simulink model "ModularDBIPSimulation"  (R2025a)
settings: Solver=FixedStepAuto  StartTime=0.0  StopTime=60  FixedStep=0.001  RelTol=1e-3
values from neighbouring files (symbols this model uses):
  A_linearized_numeric = double(subs(A_linearized,model_params,param_values))    [DBIP_CtrlStrategies.m]
  Ac = [Ac1 zeros(1,6);Ac3 Ac2]    [DBIP_CtrlStrategies.m]
  Ao = M    [DBIP_CtrlStrategies.m]
  B_linearized_numeric = double(subs(B_linearized,model_params,param_values))    [DBIP_CtrlStrategies.m]
  Bc = [Bc1;Bc2]    [DBIP_CtrlStrategies.m]
  Bo = [N P]    [DBIP_CtrlStrategies.m]
  C = eye(6)    [DBIP_SymbolicDerivation.m]
  Cc = [Cc1 Cc2]    [DBIP_CtrlStrategies.m]
  Co = Q    [DBIP_CtrlStrategies.m]
  D = [0, 0, 0, 0, 0, 0].'    [DBIP_SymbolicDerivation.m]
  Dc = zeros(1,4)    [DBIP_CtrlStrategies.m]
  Do = [R S]    [DBIP_CtrlStrategies.m]
  F = [F1 F2]    [DBIP_CtrlStrategies.m]
  theta_ref = input('Enter the desired reference theta (deg):')    [DBIP_CtrlStrategies.m]
  x0 = [deg2rad(theta_i); deg2rad(alpha_i); deg2rad(phi_i); 0; 0; 0]    [DBIP_CtrlStrategies.m]
  x2_ref = deg2rad(theta_desired)    [DBIP_CtrlStrategies.m]
  xc_o = [deg2rad(theta_i); deg2rad(alpha_i); deg2rad(phi_i); 0; 0;0;deg2rad(theta_ref)]    [DBIP_CtrlStrategies.m]
  z_o = L*(C1^-1)*y_o    [DBIP_CtrlStrategies.m]
libraries: simulink_extras x2
settings Model: Creator=young  LastModifiedBy=young
settings DataIOCC: ReturnWorkspaceOutputs=off
settings DebuggingCC: AlgebraicLoopMsg=none

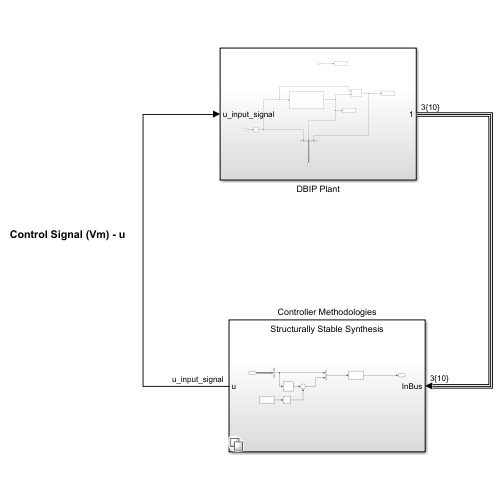
[thumbnail: Simulink's stored preview of the top-level diagram]
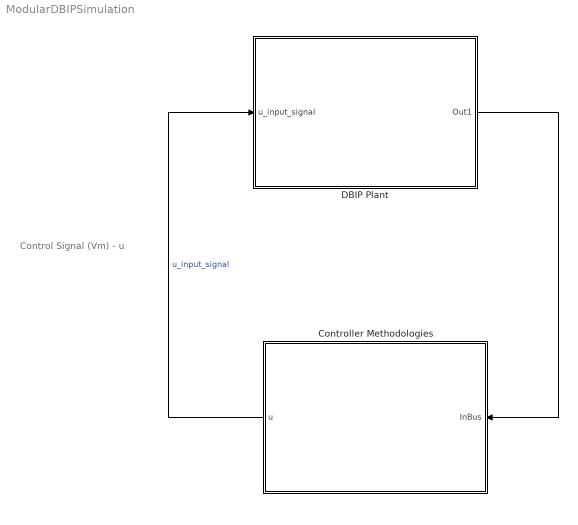
== system ModularDBIPSimulation ==
  note: Control Signal (Vm) - u
  Controller Methodologies : Subsystem  Variant=on
  DBIP Plant : Subsystem
  wires:
  Controller Methodologies/1(u) -> DBIP Plant/1(u_input_signal)  "u_input_signal"
  DBIP Plant/1(Out1) -> Controller Methodologies/1(InBus)

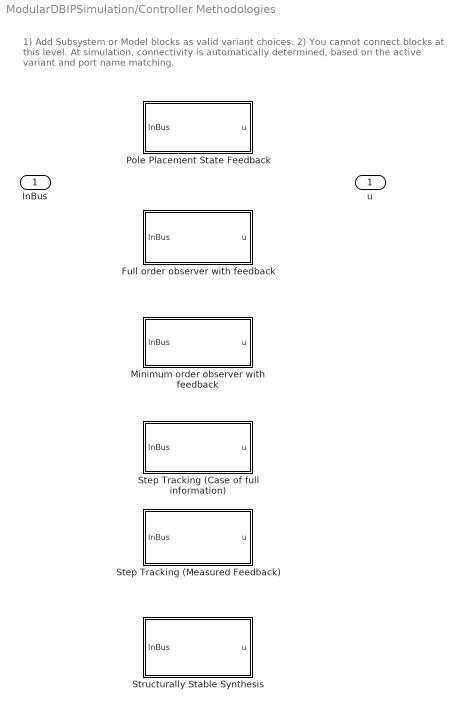
== system ModularDBIPSimulation/Controller Methodologies ==
  note: 1) Add Subsystem or Model blocks as valid variant choices.
      | 2) You cannot connect blocks at this level. At simulation, connectivity is automatically
      | determined, based on the active variant and port name matching.
  InBus : Inport
  Full order observer with feedback : Subsystem  VariantControl=control_strategy == 2
  Minimum order observer with feedback : Subsystem  VariantControl=control_strategy == 3
  Pole Placement State Feedback : Subsystem  VariantControl=control_strategy == 1
  Step Tracking (Case of full information) : Subsystem  VariantControl=control_strategy == 4
  Step Tracking (Measured Feedback) : Subsystem  VariantControl=control_strategy == 5
  Structurally Stable Synthesis : Subsystem  VariantControl=control_strategy==6
  u : Outport

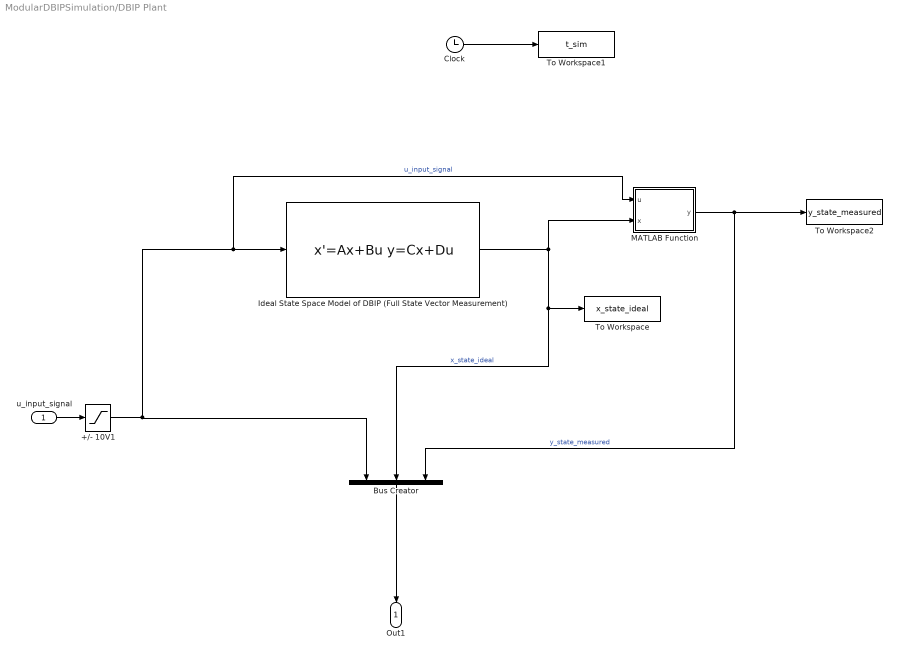
== system ModularDBIPSimulation/DBIP Plant ==
  u_input_signal : Inport
  +/- 10V1 : Saturate  UpperLimit=10  LowerLimit=-10
  Bus Creator : BusCreator  Inputs=3
  Clock : Clock
  Ideal State Space Model of DBIP (Full State Vector Measurement) : StateSpace  A=A_linearized_numeric  B=B_linearized_numeric  C=C  D=D  InitialCondition=x0
  MATLAB Function : MATLAB Function  TreatAsAtomicUnit=on
  To Workspace : ToWorkspace  VariableName=x_state_ideal  SampleTime=-1
  To Workspace1 : ToWorkspace  VariableName=t_sim  SampleTime=-1
  To Workspace2 : ToWorkspace  VariableName=y_state_measured  SampleTime=-1
  Out1 : Outport
  wires:
  MATLAB Function/1(y) -> Bus Creator/3, To Workspace2/1  "y_state_measured"
  u_input_signal/1 -> +/- 10V1/1
  Ideal State Space Model of DBIP (Full State Vector Measurement)/1 -> MATLAB Function/2(x), Bus Creator/2, To Workspace/1  "x_state_ideal"
  Bus Creator/1 -> Out1/1
  Clock/1 -> To Workspace1/1
  +/- 10V1/1 -> Ideal State Space Model of DBIP (Full State Vector Measurement)/1, MATLAB Function/1(u), Bus Creator/1  "u_input_signal"

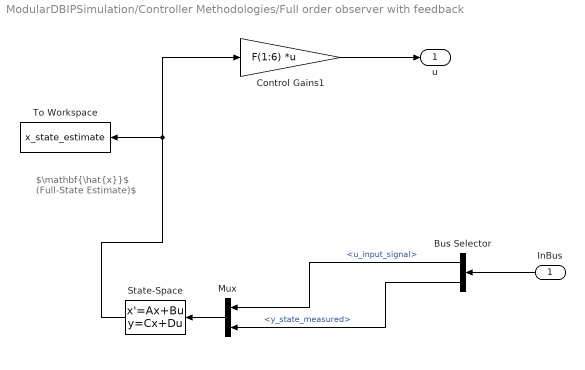
== system ModularDBIPSimulation/Controller Methodologies/Full order observer with feedback ==
  note: $\mathbf{\hat{x}}$ (Full-State Estimate)$
  InBus : Inport
  Bus Selector : BusSelector  OutputSignals=u_input_signal,y_state_measured
  Control Gains1 : Gain  Gain=F(1:6)  Multiplication=Matrix(K*u)
  Mux : Mux  Inputs=2
  State-Space : StateSpace  A=Ao  B=Bo  C=Co  D=Do  InitialCondition=z_o
  To Workspace : ToWorkspace  VariableName=x_state_estimate  SampleTime=-1
  u : Outport
  wires:
  State-Space/1 -> Control Gains1/1, To Workspace/1
  Control Gains1/1 -> u/1
  InBus/1 -> Bus Selector/1
  Bus Selector/1 -> Mux/1  "<u_input_signal>"
  Bus Selector/2 -> Mux/2  "<y_state_measured>"
  Mux/1 -> State-Space/1

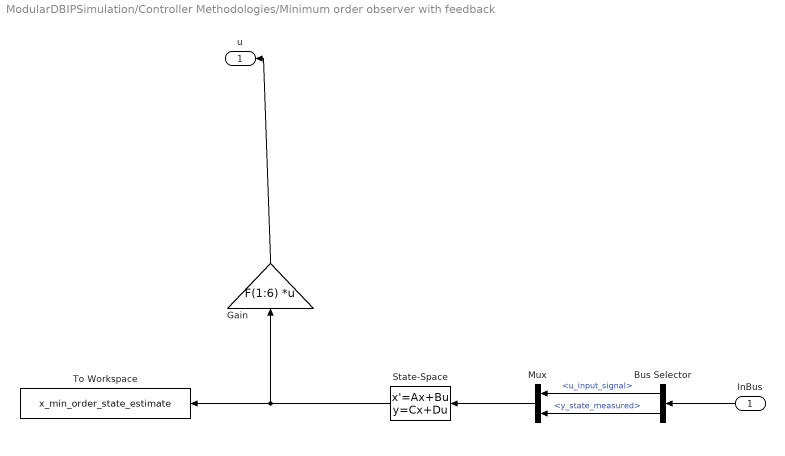
== system ModularDBIPSimulation/Controller Methodologies/Minimum order observer with feedback ==
  InBus : Inport
  Bus Selector : BusSelector  OutputSignals=u_input_signal,y_state_measured
  Gain : Gain  Gain=F(1:6)  Multiplication=Matrix(K*u)
  Mux : Mux  Inputs=2
  State-Space : StateSpace  A=Ao  B=Bo  C=Co  D=Do  InitialCondition=z_o
  To Workspace : ToWorkspace  VariableName=x_min_order_state_estimate  SampleTime=-1
  u : Outport
  wires:
  InBus/1 -> Bus Selector/1
  Gain/1 -> u/1
  State-Space/1 -> To Workspace/1, Gain/1
  Bus Selector/2 -> Mux/2  "<y_state_measured>"
  Bus Selector/1 -> Mux/1  "<u_input_signal>"
  Mux/1 -> State-Space/1

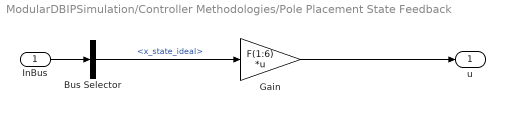
== system ModularDBIPSimulation/Controller Methodologies/Pole Placement State Feedback ==
  InBus : Inport
  Bus Selector : BusSelector  OutputSignals=x_state_ideal
  Gain : Gain  Gain=F(1:6)  Multiplication=Matrix(K*u)
  u : Outport
  wires:
  Gain/1 -> u/1
  InBus/1 -> Bus Selector/1
  Bus Selector/1 -> Gain/1  "<x_state_ideal>"

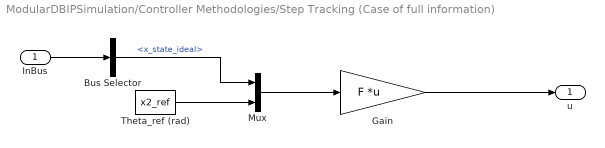
== system ModularDBIPSimulation/Controller Methodologies/Step Tracking (Case of full information) ==
  InBus : Inport
  Bus Selector : BusSelector  OutputSignals=x_state_ideal
  Gain : Gain  Gain=F  Multiplication=Matrix(K*u)
  Mux : Mux  Inputs=2
  Theta_ref (rad) : Constant  Value=x2_ref
  u : Outport
  wires:
  InBus/1 -> Bus Selector/1
  Bus Selector/1 -> Mux/1  "<x_state_ideal>"
  Theta_ref (rad)/1 -> Mux/2
  Mux/1 -> Gain/1
  Gain/1 -> u/1

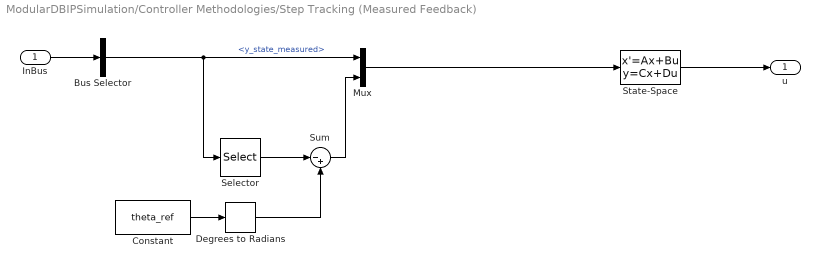
== system ModularDBIPSimulation/Controller Methodologies/Step Tracking (Measured Feedback) ==
  InBus : Inport
  Bus Selector : BusSelector  OutputSignals=y_state_measured
  Constant : Constant  Value=theta_ref
  Degrees to Radians : simulink_extras/Transformations/Degrees to Radians
  Mux : Mux  Inputs=2
  Selector : Selector  InputPortWidth=3  IndexOptions=Index vector (dialog)  Indices=[1]  OutputSizes=1
  State-Space : StateSpace  A=Ac  B=Bc  C=Cc  D=Dc  InitialCondition=xc_o
  Sum : Sum  Inputs=|-+
  u : Outport
  wires:
  InBus/1 -> Bus Selector/1
  Constant/1 -> Degrees to Radians/1
  Bus Selector/1 -> Mux/1, Selector/1  "<y_state_measured>"
  Degrees to Radians/1 -> Sum/2
  Mux/1 -> State-Space/1
  State-Space/1 -> u/1
  Selector/1 -> Sum/1
  Sum/1 -> Mux/2

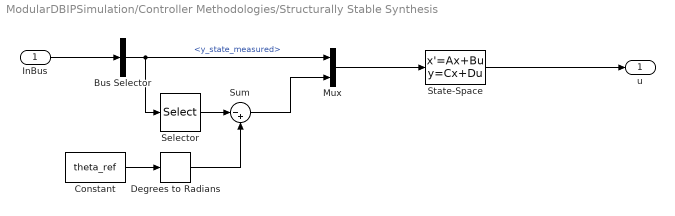
== system ModularDBIPSimulation/Controller Methodologies/Structurally Stable Synthesis ==
  InBus : Inport
  Bus Selector : BusSelector  OutputSignals=y_state_measured
  Constant : Constant  Value=theta_ref
  Degrees to Radians : simulink_extras/Transformations/Degrees to Radians
  Mux : Mux  Inputs=2
  Selector : Selector  InputPortWidth=3  IndexOptions=Index vector (dialog)  Indices=[1]  OutputSizes=1
  State-Space : StateSpace  A=Ac  B=Bc  C=Cc  D=Dc  InitialCondition=xc_o
  Sum : Sum  Inputs=|-+
  u : Outport
  wires:
  State-Space/1 -> u/1
  InBus/1 -> Bus Selector/1
  Constant/1 -> Degrees to Radians/1
  Mux/1 -> State-Space/1
  Bus Selector/1 -> Selector/1, Mux/1  "<y_state_measured>"
  Selector/1 -> Sum/1
  Degrees to Radians/1 -> Sum/2
  Sum/1 -> Mux/2

== matlab function ModularDBIPSimulation/DBIP Plant/MATLAB Function ==
  data: u input; x input; y output
function y = CxDu(u,x)
C = [1 0 0 0 0 0;
     0 1 0 0 0 0;
     0 0 1 0 0 0];
D = [0;0;0];
y = C*x+D*u;
